simulink model "Simulation_DOA_rearanged_2020a"  (R2020a)
settings: Solver=ode4  StartTime=0.0  StopTime=0.03  RelTol=1e-3
values from neighbouring files (symbols this model uses):
  f_range = [20e3 45e3]    [Init.m]
  FFT_LENGTH = 256    [Init.m]
  noise_on_off = false    [Init.m]
  noise_type = 1    [Init.m]
  Sampling_rate = 256e3    (= 256000)    [Init.m]
undefined symbols (not defined in the file or in its folder): Coeff_han, runSim
libraries: dspsigops x29, dspsrcs4 x16, dsphdlmathfun x4, dsphdlxfrm x4, simulink x2, hdlsllib x1
(part 2 of 2)

== system Simulation_DOA_rearanged_2020a/Signal Trigger/Fenetrage ==
  Valid_in : Inport
  Enable : Inport  Port=2
  Constant : Constant  Value=0  OutDataTypeStr=uint16  SampleTime=1/Sampling_rate
  Direct Lookup Table (n-D) : LookupNDDirect  NumberOfTableDimensions=1  Table=Coeff_han  DiagnosticForOutOfRangeInput=Error  TableMin=[0]  TableDataTypeStr=fixdt(0,9,8)
  Scope : Scope
  Subsystem : Subsystem
  Switch : Switch  Threshold=FFT_LENGTH  OutMin=[0]  OutMax=[511]  OutDataTypeStr=uint16
  coeff : Outport
  wires:
  Direct Lookup Table (n-D)/1 -> coeff/1
  Valid_in/1 -> Subsystem/1(Reset)
  Switch/1 -> Direct Lookup Table (n-D)/1
  Subsystem/1(Count) -> Switch/2, Switch/3, Scope/1
  Constant/1 -> Switch/1
  Enable/1 -> Subsystem/2(Enable)

== system Simulation_DOA_rearanged_2020a/Subsystem4/Triggered Subsystem1 ==
  Somme : Inport
  " Valeur Max" : Inport  Port=2
  SNR_Threshold : Inport  Port=3
  Trigger : TriggerPort  VariantControl=Variant
  Data Type Conversion : DataTypeConversion  OutDataTypeStr=fixdt(1,27,8)
  Divide : Product  Inputs=*/  RndMeth=Zero  SaturateOnIntegerOverflow=on
  Relational Operator : RelationalOperator  OutDataTypeStr=boolean  RndMeth=Simplest
  SNR check : Outport  InitialOutput=[0]  VectorParamsAs1DForOutWhenUnconnected=off
  Debug : Outport  Port=2  InitialOutput=[0]  VectorParamsAs1DForOutWhenUnconnected=off
  wires:
  Relational Operator/1 -> SNR check/1
  SNR_Threshold/1 -> Data Type Conversion/1
  " Valeur Max"/1 -> Divide/2
  Somme/1 -> Divide/1
  Data Type Conversion/1 -> Relational Operator/2
  Divide/1 -> Relational Operator/1, Debug/1

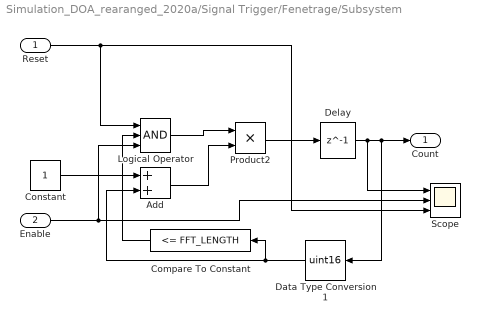
== system Simulation_DOA_rearanged_2020a/Signal Trigger/Fenetrage/Subsystem ==
  Reset : Inport
  Enable : Inport  Port=2
  Add : Sum
  Compare To Constant : simulink/Logic and Bit Operations/Compare To Constant  relop=<=  const=FFT_LENGTH  OutDataTypeStr=boolean
  Constant : Constant  OutDataTypeStr=Inherit: Inherit via back propagation  SampleTime=1/256000
  Data Type Conversion1 : DataTypeConversion  OutDataTypeStr=uint16  RndMeth=Nearest
  Delay : Delay  DelayLength=1  InitialCondition=0  UseCircularBuffer=on
  Logical Operator : Logic  Inputs=3  AllPortsSameDT=off  OutDataTypeStr=boolean
  Product2 : Product  OutDataTypeStr=uint16
  Scope : Scope  NumInputPorts=3
  Count : Outport  VectorParamsAs1DForOutWhenUnconnected=off
  wires:
  Delay/1 -> Scope/1, Count/1, Data Type Conversion1/1
  Product2/1 -> Delay/1
  Data Type Conversion1/1 -> Add/2, Compare To Constant/1
  Reset/1 -> Scope/3, Logical Operator/1
  Compare To Constant/1 -> Logical Operator/2
  Logical Operator/1 -> Product2/1
  Add/1 -> Product2/2
  Constant/1 -> Add/1
  Enable/1 -> Scope/2, Logical Operator/3
